simulink model "MandS_Project_Pistol_Research_Paper"  (R2023b)
settings: Solver=VariableStepAuto  StartTime=0.0  StopTime=2  RelTol=1e-3
model workspace (MAT data in the model file):
  Chx = Simulink.Parameter
  Chx.Value = 163000
  Chx.DataType = 'auto'
  Chx.DocUnits = 'Ns/m'
  Chx.Complexity = 'real'
  Chx.Dimensions = [1 1]
  Chy = Simulink.Parameter
  Chy.Value = 123000
  Chy.DataType = 'auto'
  Chy.DocUnits = 'Ns/m'
  Chy.Complexity = 'real'
  Chy.Dimensions = [1 1]
  I = Simulink.Parameter
  I.Value = 0.00625
  I.DataType = 'auto'
  I.DocUnits = 'kgm^2'
  I.Complexity = 'real'
  I.Dimensions = [1 1]
  Khx = Simulink.Parameter
  Khx.Value = 1000
  Khx.DataType = 'auto'
  Khx.DocUnits = 'N/m'
  Khx.Complexity = 'real'
  Khx.Dimensions = [1 1]
  Khy = Simulink.Parameter
  Khy.Value = 1000
  Khy.DataType = 'auto'
  Khy.DocUnits = 'N/m'
  Khy.Complexity = 'real'
  Khy.Dimensions = [1 1]
  L2 = Simulink.Parameter
  L2.Value = 150
  L2.DataType = 'auto'
  L2.DocUnits = 'cm'
  L2.Complexity = 'real'
  L2.Dimensions = [1 1]
  L3 = Simulink.Parameter
  L3.Value = 60
  L3.DataType = 'auto'
  L3.DocUnits = 'cm'
  L3.Complexity = 'real'
  L3.Dimensions = [1 1]
  c1 = Simulink.Parameter
  c1.Value = 1000
  c1.DataType = 'auto'
  c1.DocUnits = 'Ns/m'
  c1.Complexity = 'real'
  c1.Dimensions = [1 1]
  c2 = Simulink.Parameter
  c2.Value = 1000
  c2.DataType = 'auto'
  c2.DocUnits = 'Ns/m'
  c2.Complexity = 'real'
  c2.Dimensions = [1 1]
  k1 = Simulink.Parameter
  k1.Value = 2276.65
  k1.DataType = 'auto'
  k1.DocUnits = 'N/m'
  k1.Complexity = 'real'
  k1.Dimensions = [1 1]
  k2 = Simulink.Parameter
  k2.Value = 0
  k2.DataType = 'auto'
  k2.DocUnits = 'N/m'
  k2.Complexity = 'real'
  k2.Dimensions = [1 1]
  m = Simulink.Parameter
  m.Value = 1
  m.DataType = 'auto'
  m.DocUnits = 'kg'
  m.Complexity = 'real'
  m.Dimensions = [1 1]
  m1 = Simulink.Parameter
  m1.Value = 0.5
  m1.DataType = 'auto'
  m1.DocUnits = 'kg'
  m1.Complexity = 'real'
  m1.Dimensions = [1 1]
  s = Simulink.Parameter
  s.Value = 3
  s.DataType = 'auto'
  s.DocUnits = 'cm'
  s.Complexity = 'real'
  s.Dimensions = [1 1]
  z = Simulink.Parameter
  z.Value = 1
  z.DataType = 'auto'
  z.DocUnits = 'cm'
  z.Complexity = 'real'
  z.Dimensions = [1 1]
settings Model: Creator=Sarmad Ahmad  LastModifiedBy=Sarmad Ahmad
settings DebuggingCC: IgnoredZcDiagnostic=none

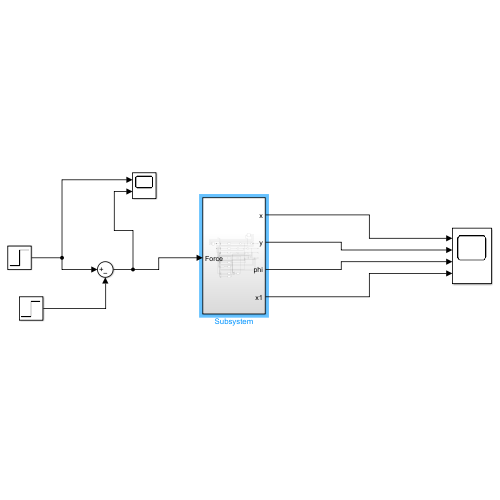
[thumbnail: Simulink's stored preview of the top-level diagram]
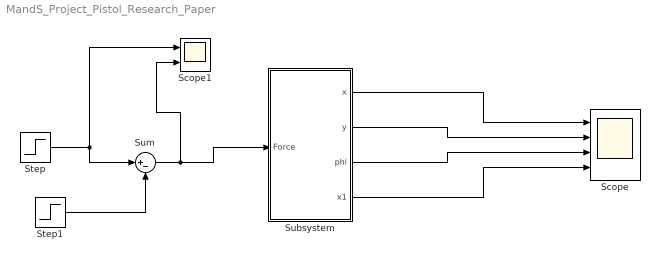
== system MandS_Project_Pistol_Research_Paper ==
  Scope : Scope  NumInputPorts=4
  Scope1 : Scope  NumInputPorts=2
  Step : Step  After=2200  SampleTime=0
  Step1 : Step  Time=1.1  After=2200  SampleTime=0
  Subsystem : Subsystem
  Sum : Sum  Inputs=|+-
  wires:
  Subsystem/1(x) -> Scope/1
  Subsystem/2(y) -> Scope/2
  Subsystem/3(phi) -> Scope/3
  Subsystem/4(x1) -> Scope/4
  Step/1 -> Sum/1, Scope1/1
  Step1/1 -> Sum/2
  Sum/1 -> Scope1/2, Subsystem/1(Force)

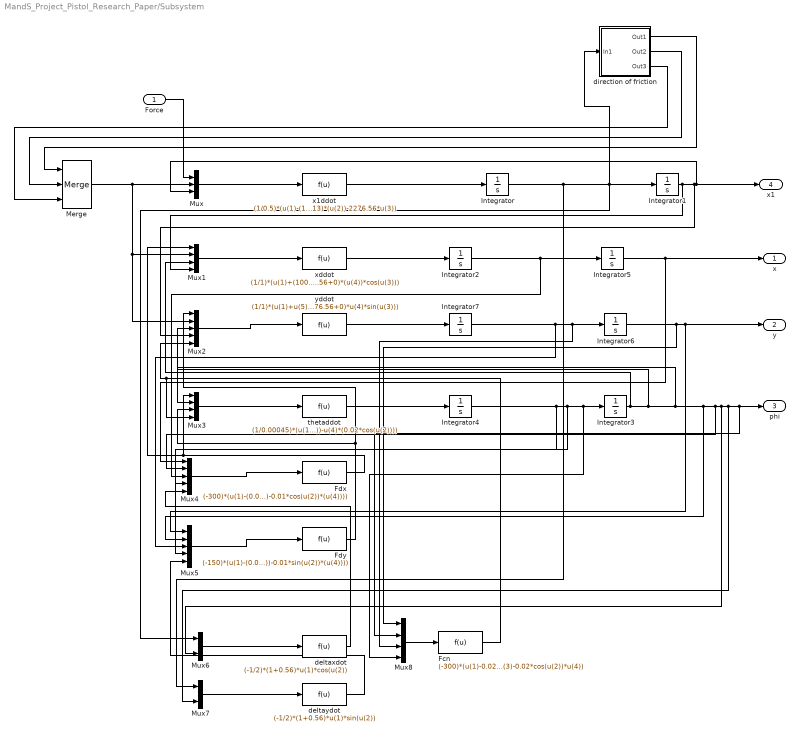
== system MandS_Project_Pistol_Research_Paper/Subsystem ==
  Force : Inport
  Fcn : Fcn  Expr=(-300)*(u(1)-0.02*sin(u(2))-1.55)-10.13*(u(3)-0.02*cos(u(2))*u(4))
  Fdx : Fcn  Expr=(-300)*(u(1)-(0.03*cos(u(2))-0.01*sin(u(2))+0.6))-3*(u(3)-(-u(5)-0.03*sin(u(2))*(u(4))-0.01*cos(u(2))*(u(4))))
  Fdy : Fcn  Expr=(-150)*(u(1)-(0.03*sin(u(2))+0.01*cos(u(2))+1.5))-5*(u(3)-(-u(5)+0.03*cos(u(2))*(u(4))-0.01*sin(u(2))*(u(4))))
  Integrator{,1..7} (8 alike) : Integrator
  Merge : Merge  Inputs=3
  Mux : Mux  Inputs=3
  Mux1 : Mux
  Mux2 : Mux  Inputs=5
  Mux3 : Mux
  Mux4 : Mux  Inputs=5
  Mux5 : Mux  Inputs=5
  Mux6 : Mux  Inputs=2
  Mux7 : Mux  Inputs=2
  Mux8 : Mux
  deltaxdot : Fcn  Expr=(-1/2)*(1+0.56)*u(1)*cos(u(2))
  deltaydot : Fcn  Expr=(-1/2)*(1+0.56)*u(1)*sin(u(2))
  direction of friction : Subsystem
  thetaddot : Fcn  Expr=(1/0.00045)*(u(1)*(0.03*sin(u(2))+0.01*cos(u(2)))-u(3)*(0.03*cos(u(2))-0.01*sin(u(2)))-u(4)*(0.02*cos(u(2))))
  x1ddot : Fcn  Expr=(1/0.5)*(u(1)-(100.13+100.13)*(u(2))-2276.56*u(3))
  xddot : Fcn  Expr=(1/1)*(u(1)+(100.13+100.13)*u(2)*cos(u(3))+(2276.56+0)*(u(4))*cos(u(3)))
  yddot : Fcn  Expr=(1/1)*(u(1)+u(5)+(100.13+100.13)*u(2)*sin(u(3))+(2276.56+0)*u(4)*sin(u(3)))
  x : Outport
  y : Outport  Port=2
  phi : Outport  Port=3
  x1 : Outport  Port=4
  wires:
  Mux1/1 -> xddot/1
  Integrator4/1 -> Mux4/4, Mux5/4, Mux8/4, Integrator3/1
  Mux/1 -> x1ddot/1
  Mux2/1 -> yddot/1
  Force/1 -> Mux/1
  Integrator3/1 -> Mux1/3, Mux2/3, Mux3/2, Mux5/2, Mux6/2, Mux7/2, Mux8/2, phi/1, Mux4/2
  Integrator1/1 -> Mux1/4, Mux2/4, x1/1, Mux/3
  xddot/1 -> Integrator2/1
  Integrator2/1 -> Mux4/3, Integrator5/1
  Mux4/1 -> Fdx/1
  Fdx/1 -> Mux3/1, Mux1/1
  Integrator/1 -> Mux7/1, Mux6/1, direction of friction/1(In1), Integrator1/1
  Mux3/1 -> thetaddot/1
  Integrator7/1 -> Mux5/3, Mux8/3, Integrator6/1
  Mux5/1 -> Fdy/1
  Fdy/1 -> Mux3/3, Mux2/1
  Integrator5/1 -> x/1, Mux4/1
  yddot/1 -> Integrator7/1
  Integrator6/1 -> Mux8/1, y/1, Mux5/1
  x1ddot/1 -> Integrator/1
  thetaddot/1 -> Integrator4/1
  Merge/1 -> Mux2/2, Mux1/2, Mux/2
  direction of friction/1(Out1) -> Merge/1
  direction of friction/2(Out2) -> Merge/2
  direction of friction/3(Out3) -> Merge/3
  Mux6/1 -> deltaxdot/1
  Mux7/1 -> deltaydot/1
  deltaxdot/1 -> Mux4/5
  deltaydot/1 -> Mux5/5
  Mux8/1 -> Fcn/1
  Fcn/1 -> Mux3/4, Mux2/5

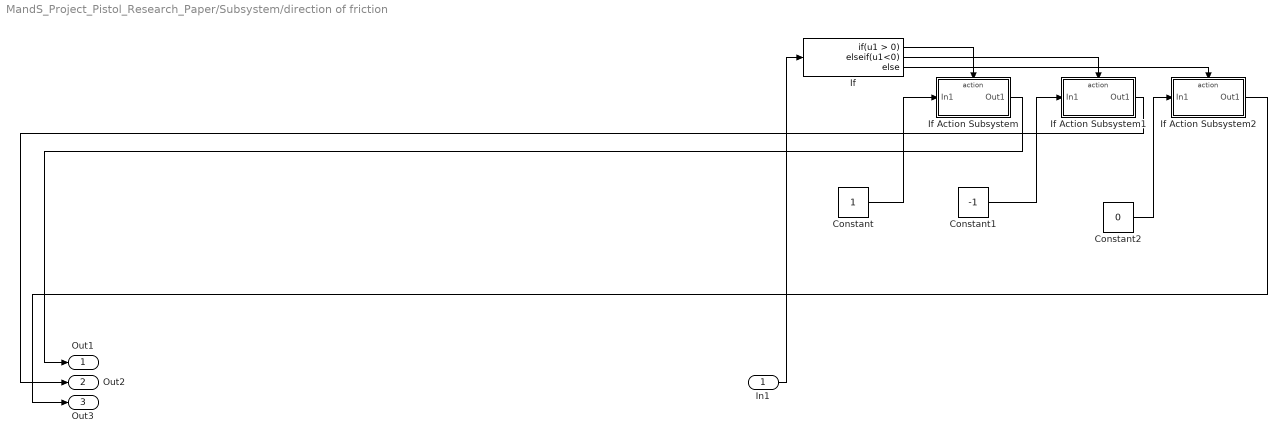
== system MandS_Project_Pistol_Research_Paper/Subsystem/direction of friction ==
  In1 : Inport
  Constant : Constant
  Constant1 : Constant  Value=-1
  Constant2 : Constant  Value=0
  If : If  ElseIfExpressions=u1<0  ZeroCross=off
  If Action Subsystem : Subsystem  TreatAsAtomicUnit=on
  If Action Subsystem1 : Subsystem  TreatAsAtomicUnit=on
  If Action Subsystem2 : Subsystem  TreatAsAtomicUnit=on
  Out1 : Outport
  Out2 : Outport  Port=2
  Out3 : Outport  Port=3
  wires:
  If/1 -> If Action Subsystem/Action
  Constant1/1 -> If Action Subsystem1/1(In1)
  In1/1 -> If/1
  If/2 -> If Action Subsystem1/Action
  If Action Subsystem2/1(Out1) -> Out3/1
  Constant/1 -> If Action Subsystem/1(In1)
  If Action Subsystem1/1(Out1) -> Out2/1
  If/3 -> If Action Subsystem2/Action
  Constant2/1 -> If Action Subsystem2/1(In1)
  If Action Subsystem/1(Out1) -> Out1/1

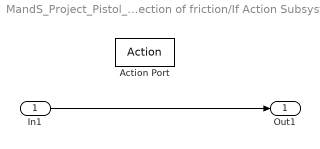
== system MandS_Project_Pistol_Research_Paper/Subsystem/direction of friction/If Action Subsystem ==
  In1 : Inport
  Action Port : ActionPort  ActionPortLabel=if(u1 > 0)
  Out1 : Outport
  wires:
  In1/1 -> Out1/1

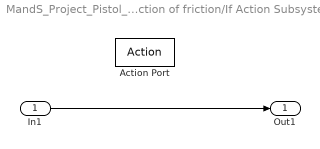
== system MandS_Project_Pistol_Research_Paper/Subsystem/direction of friction/If Action Subsystem1 ==
  In1 : Inport
  Action Port : ActionPort  ActionPortLabel=elseif(u1<0)
  Out1 : Outport
  wires:
  In1/1 -> Out1/1

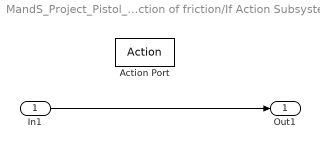
== system MandS_Project_Pistol_Research_Paper/Subsystem/direction of friction/If Action Subsystem2 ==
  In1 : Inport
  Action Port : ActionPort  ActionPortLabel=else
  Out1 : Outport
  wires:
  In1/1 -> Out1/1
